simulink model "Hybrid_Flight_Lib"  (R2025a)
settings: Solver=VariableStepAuto  StartTime=0.0  StopTime=10.0  RelTol=1e-3
settings Model: Creator=maxal  LastModifiedBy=maxal

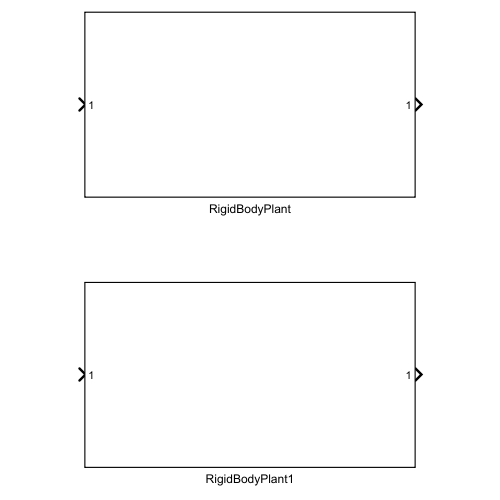
[thumbnail: Simulink's stored preview of the top-level diagram]
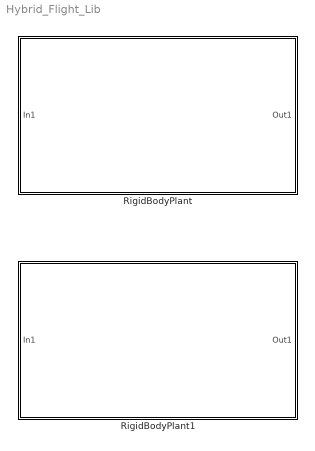
== system Hybrid_Flight_Lib ==
  RigidBodyPlant : Subsystem
  RigidBodyPlant1 : Subsystem

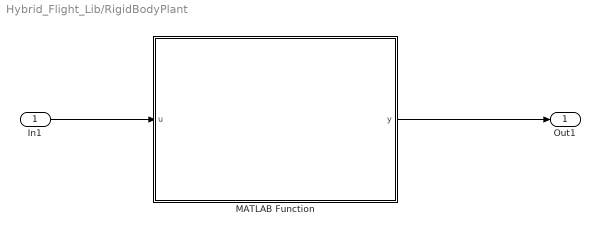
== system Hybrid_Flight_Lib/RigidBodyPlant ==
  In1 : Inport
  MATLAB Function : MATLAB Function  TreatAsAtomicUnit=on  mask{mass=0, I_body=0}
  Out1 : Outport
  wires:
  In1/1 -> MATLAB Function/1(u)
  MATLAB Function/1(y) -> Out1/1

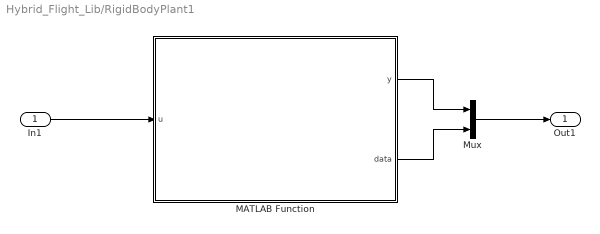
== system Hybrid_Flight_Lib/RigidBodyPlant1 ==
  In1 : Inport
  MATLAB Function : MATLAB Function  TreatAsAtomicUnit=on  mask{mass=0, I_body=0}
  Mux : Mux  Inputs=2
  Out1 : Outport
  wires:
  In1/1 -> MATLAB Function/1(u)
  Mux/1 -> Out1/1
  MATLAB Function/2(data) -> Mux/2
  MATLAB Function/1(y) -> Mux/1

== matlab function Hybrid_Flight_Lib/RigidBodyPlant/MATLAB Function ==
  data: u input; y output
% function [y,data] = fcn(u)
function y  = fcn(u)
persistent plant xRB
if isempty(plant)
    % cfg = AeroFlex.cfg.defaultConfig;
    cfg = nominalConfig;
    % I = reshape(I_body,3,3);  
    plant = AeroFlex.sim.FlexCoupler(cfg, mass, I_body);
    % xRB   = zeros(10,1);                    % q euler etc.
end
xRB = u;
wgust = 0;                                 % connect later
[xRB,~] = plant.step(xRB, zeros(1,plant.wing.nq), wgust);
y = xRB;

== matlab function Hybrid_Flight_Lib/RigidBodyPlant1/MATLAB Function ==
  data: u input; y output; data output
function [y,data] = fcn(u)
persistent plant xRB
if isempty(plant)
    cfg = AeroFlex.cfg.defaultConfig;
    I = reshape(I_body,3,3);  
    plant = AeroFlex.sim.FlexCoupler(cfg, mass, I_body);
    xRB   = zeros(10,1);                    % q euler etc.
end
wgust = 0;                                 % connect later
[xRB,~] = plant.step(xRB, zeros(1,plant.wing.nq), wgust);
y = xRB;
